simulink model "powersupply_1jan_old_top"  (R2015b)
settings: Solver=ode45  StartTime=0.0  StopTime=20*T_mach  MaxStep=4e-7  MinStep=1e-8  RelTol=1e-3
values from neighbouring files (symbols this model uses):
  c2_val = (1-V_ref/Vd_val)/(8*v2_ripple*l2_val*f_sw^2)    (= 0.0001)    [PowerSupplyScript.m]    (also in master_conv.m; master_conv2.m = 6.25e-07; matlab.mat = 1e-05; normal_buck_comparison.m = 1e-05)
  Cs = (Cs_min + Cs_max) / 2    (= 1.43223295455e-05)    [PowerSupplyScript.m]    (also in QdSnubber.m = (Cs_min + Cs_max) / 2; master_conv2.m = 3.126125e-05; matlab.mat = 2.98407954545e-05)
  delay_load = t1    (= 6e-06)    [PowerSupplyScript.m]    (also in master_conv.m; master_conv2.m; matlab.mat)
  delayVC = 2e-3    (= 0.002)    [PowerSupplyScript.m]    (also in master_conv.m = 0.001; master_conv2.m = 0; matlab.mat = 0)
  den_c1 =     [matlab.mat]
  den_c2 =     [matlab.mat]
  duty_inv = 100 - duty    (= 90)    [PowerSupplyScript.m]    (also in master_conv.m; master_conv2.m; matlab.mat)
  duty_load = (t2-t1)/T_mach*100    (= 7)    [PowerSupplyScript.m]    (also in master_conv.m; master_conv2.m; matlab.mat)
  f_sw = 50e3    (= 50000)    [PowerSupplyScript.m]    (also in master_conv.m; master_conv2.m; matlab.mat)
  frq_dc = 50    [master_conv2.m]    (also in matlab.mat = 10)
  I_ref = 10    [PowerSupplyScript.m]    (also in master_conv.m; master_conv2.m; matlab.mat)
  l1_val = Vo1*(Vd_val-Vo1)/(delta_i1*f_sw*Vd_val)    (= 0.00181818181818)    [PowerSupplyScript.m]    (also in master_conv.m = 0.000181818181818; master_conv2.m; matlab.mat; poles_locus.m = l1_val_bak)
  l2_val = 2.5*r_val*(Vd_val-V_ref)/(f_sw*Vd_val)    (= 1.36363636364e-05)    [PowerSupplyScript.m]    (also in master_conv.m; master_conv2.m = 0.00218181818182; matlab.mat = 0.002; poles_locus.m = l2_val_bak)
  num_c1 =     [matlab.mat]
  num_c2 =     [matlab.mat]
  r_val = 1    [PowerSupplyScript.m]    (also in master_conv.m; master_conv2.m; matlab.mat)
  rc2_val = 0.0001    [PowerSupplyScript.m]    (also in master_conv.m; master_conv2.m; matlab.mat)
  rl1_val = 0.0002    [PowerSupplyScript.m]    (also in master_conv.m; master_conv2.m; matlab.mat)
  rl2_val = 0.0001    [PowerSupplyScript.m]    (also in master_conv.m; master_conv2.m; matlab.mat)
  Rs = V_ref / I_ref    (= 8)    [PowerSupplyScript.m]    (also in QdSnubber.m = V_ref / I_ref; master_conv2.m; matlab.mat)
  t2 = duty * T_mach / 100    (= 2e-05)    [PowerSupplyScript.m]    (also in master_conv.m; master_conv2.m; matlab.mat)
  T_mach = 200e-6    (= 0.0002)    [PowerSupplyScript.m]    (also in master_conv.m; master_conv2.m; matlab.mat)
  V_ref = 80    [PowerSupplyScript.m]    (also in master_conv.m; master_conv2.m; matlab.mat)
  Vd_val = 110    [PowerSupplyScript.m]    (also in master_conv.m; master_conv2.m; matlab.mat)
libraries: powerlib x86, simulink x10, powerlib_meascontrol x8, simulink_extras x6
(part 2 of 2)

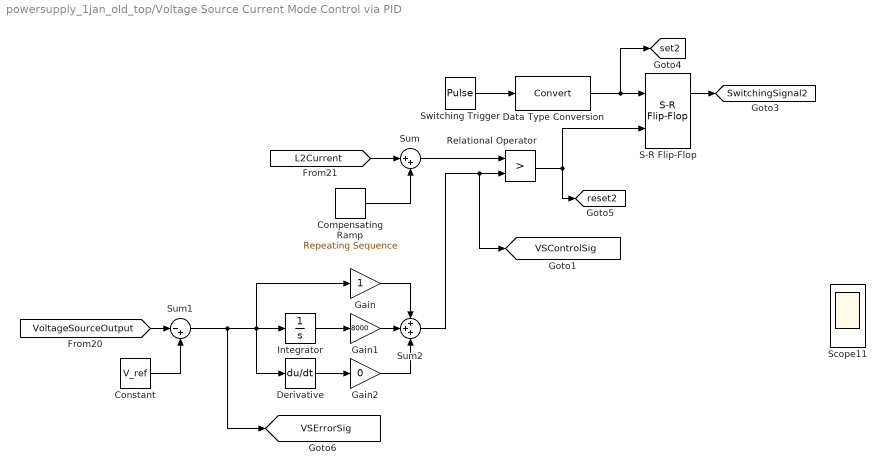
== system powersupply_1jan_old_top/Voltage Source Current Mode Control via PID ==
  Compensating Ramp : simulink/Sources/Repeating Sequence  rep_seq_t=[0 1/f_sw]  rep_seq_y=[0 80]
  Constant : Constant  Value=V_ref
  Data Type Conversion : DataTypeConversion
  Derivative : Derivative
  Gain : Gain
  Gain1 : Gain  Gain=8000
  Gain2 : Gain  Gain=0
  Integrator : Integrator
  Relational Operator : RelationalOperator  Operator=>  OutDataTypeStr=boolean
  S-R Flip-Flop : simulink_extras/Flip Flops/S-R Flip-Flop  initial_condition=0
  Scope11 : Scope  NumInputPorts=4
  Sum : Sum  Inputs=|++
  Sum1 : Sum  Inputs=|-+
  Sum2 : Sum  Inputs=+++
  Switching Trigger : DiscretePulseGenerator  PulseType=Time based  Period=1/f_sw  PulseWidth=5
  tag scope: SwitchingSignal2=global, VSControlSig=global, VSErrorSig=global, reset2=global, set2=global
  wires:
  Switching Trigger/1 -> Data Type Conversion/1
  Data Type Conversion/1 -> S-R Flip-Flop/1, [set2]
  Relational Operator/1 -> S-R Flip-Flop/2, [reset2]
  S-R Flip-Flop/1 -> [SwitchingSignal2]
  [L2Current] -> Sum/1
  Compensating Ramp/1 -> Sum/2
  Sum/1 -> Relational Operator/1
  [VoltageSourceOutput] -> Sum1/1
  Constant/1 -> Sum1/2
  Sum1/1 -> [VSErrorSig], Derivative/1, Gain/1, Integrator/1
  Integrator/1 -> Gain1/1
  Gain1/1 -> Sum2/2
  Gain/1 -> Sum2/1
  Sum2/1 -> [VSControlSig], Relational Operator/2
  Derivative/1 -> Gain2/1
  Gain2/1 -> Sum2/3

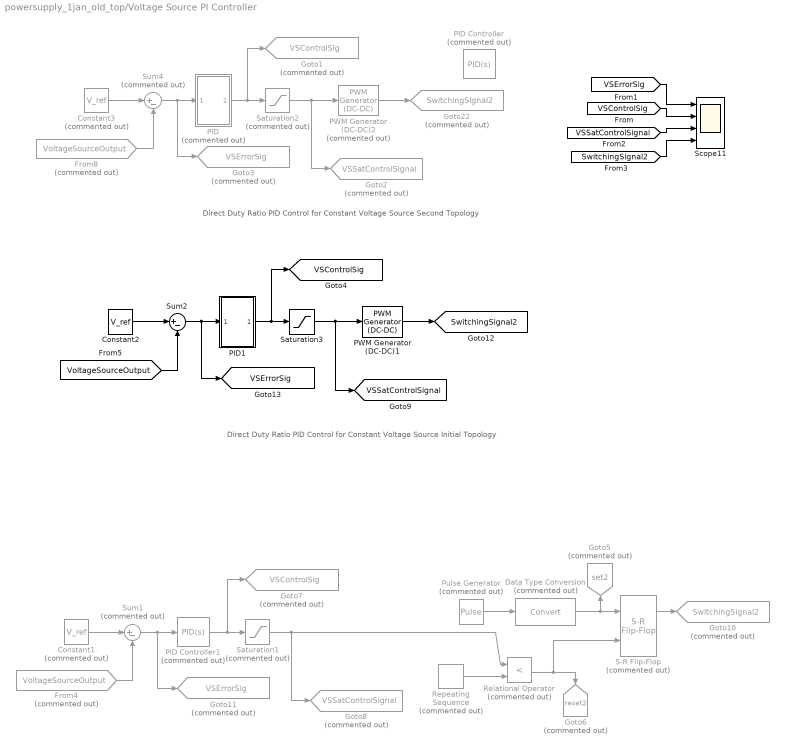
== system powersupply_1jan_old_top/Voltage Source PI Controller ==
  note: Direct Duty Ratio PID Control for Constant Voltage Source
      | Second Topology
  note: Direct Duty Ratio PID Control for Constant Voltage Source
      | Initial Topology
  Constant1 : Constant  Commented=on  Value=V_ref
  Constant2 : Constant  Value=V_ref
  Constant3 : Constant  Commented=on  Value=V_ref
  Data Type Conversion : DataTypeConversion  Commented=on
  From4 : From  Commented=on  GotoTag=VoltageSourceOutput  TagVisibility=global
  From8 : From  Commented=on  GotoTag=VoltageSourceOutput  TagVisibility=global
  Goto1 : Goto  Commented=on  GotoTag=VSControlSig  TagVisibility=global
  Goto10 : Goto  Commented=on  GotoTag=SwitchingSignal2  TagVisibility=global
  Goto11 : Goto  Commented=on  GotoTag=VSErrorSig  TagVisibility=global
  Goto2 : Goto  Commented=on  GotoTag=VSSatControlSignal  TagVisibility=global
  Goto22 : Goto  Commented=on  GotoTag=SwitchingSignal2  TagVisibility=global
  Goto3 : Goto  Commented=on  GotoTag=VSErrorSig  TagVisibility=global
  Goto5 : Goto  Commented=on  GotoTag=set2  TagVisibility=global
  Goto6 : Goto  Commented=on  GotoTag=reset2  TagVisibility=global
  Goto7 : Goto  Commented=on  GotoTag=VSControlSig  TagVisibility=global
  Goto8 : Goto  Commented=on  GotoTag=VSSatControlSignal  TagVisibility=global
  PID : Subsystem  Commented=on
  PID Controller : simulink/Continuous/PID Controller  Commented=on  Controller=PID  TimeDomain=Continuous-time  SampleTime=-1  IntegratorMethod=Forward Euler  FilterMethod=Forward Euler  Form=Parallel  UseFilter=on  ControllerParametersSource=internal  P=5  I=0  D=1  N=100000  InitialConditionSource=internal  InitialConditionForIntegrator=0  InitialConditionForFilter=0  ExternalReset=none  LimitOutput=off  UpperSaturationLimit=inf  LowerSaturationLimit=-inf  LinearizeAsGain=on  AntiWindupMode=none  Kb=1  TrackingMode=off  Kt=1  PParamMin=[]  PParamMax=[]  IParamMin=[]  IParamMax=[]  DParamMin=[]  DParamMax=[]  NParamMin=[]  NParamMax=[]  KbParamMin=[]  KbParamMax=[]  KtParamMin=[]  KtParamMax=[]  POutMin=[]  POutMax=[]  IOutMin=[]  IOutMax=[]  DOutMin=[]  DOutMax=[]  NOutMin=[]  NOutMax=[]  KbOutMin=[]  KbOutMax=[]  KtOutMin=[]  KtOutMax=[]  IntegratorOutMin=[]  IntegratorOutMax=[]  FilterOutMin=[]  FilterOutMax=[]  SumOutMin=[]  SumOutMax=[]  SumI1OutMin=[]  SumI1OutMax=[]  SumI2OutMin=[]  SumI2OutMax=[]  SumI3OutMin=[]  SumI3OutMax=[]  SumDOutMin=[]  SumDOutMax=[]  SaturationOutMin=[]  SaturationOutMax=[]  IntegratorContinuousStateAttributes=''  IntegratorStateMustResolveToSignalObject=off  IntegratorRTWStateStorageClass=Auto  FilterContinuousStateAttributes=''  FilterStateMustResolveToSignalObject=off  FilterRTWStateStorageClass=Auto  DifferentiatorICPrevScaledInput=0  DifferentiatorOutMin=[]  DifferentiatorOutMax=[]
  PID Controller1 : simulink/Continuous/PID Controller  Commented=on  Controller=PID  TimeDomain=Continuous-time  SampleTime=-1  IntegratorMethod=Forward Euler  FilterMethod=Forward Euler  Form=Parallel  UseFilter=on  ControllerParametersSource=internal  P=0.0189788446035745  I=203.066732311021  D=4.39436806782284e-07  N=6149446.46601847  InitialConditionSource=internal  InitialConditionForIntegrator=0  InitialConditionForFilter=0  ExternalReset=none  LimitOutput=off  UpperSaturationLimit=inf  LowerSaturationLimit=-inf  LinearizeAsGain=on  AntiWindupMode=none  Kb=1  TrackingMode=off  Kt=1  PParamMin=[]  PParamMax=[]  IParamMin=[]  IParamMax=[]  DParamMin=[]  DParamMax=[]  NParamMin=[]  NParamMax=[]  KbParamMin=[]  KbParamMax=[]  KtParamMin=[]  KtParamMax=[]  POutMin=[]  POutMax=[]  IOutMin=[]  IOutMax=[]  DOutMin=[]  DOutMax=[]  NOutMin=[]  NOutMax=[]  KbOutMin=[]  KbOutMax=[]  KtOutMin=[]  KtOutMax=[]  IntegratorOutMin=[]  IntegratorOutMax=[]  FilterOutMin=[]  FilterOutMax=[]  SumOutMin=[]  SumOutMax=[]  SumI1OutMin=[]  SumI1OutMax=[]  SumI2OutMin=[]  SumI2OutMax=[]  SumI3OutMin=[]  SumI3OutMax=[]  SumDOutMin=[]  SumDOutMax=[]  SaturationOutMin=[]  SaturationOutMax=[]  IntegratorContinuousStateAttributes=''  IntegratorStateMustResolveToSignalObject=off  IntegratorRTWStateStorageClass=Auto  FilterContinuousStateAttributes=''  FilterStateMustResolveToSignalObject=off  FilterRTWStateStorageClass=Auto  DifferentiatorICPrevScaledInput=0  DifferentiatorOutMin=[]  DifferentiatorOutMax=[]
  PID1 : Subsystem
  PWM Generator (DC-DC)1 : powerlib_meascontrol/Pulse & Signal Generators/PWM Generator (DC-DC)  Fsw=f_sw  Ts=0
  PWM Generator (DC-DC)2 : powerlib_meascontrol/Pulse & Signal Generators/PWM Generator (DC-DC)  Commented=on  Fsw=f_sw  Ts=0
  Pulse Generator : DiscretePulseGenerator  Commented=on  PulseType=Time based  Period=1/f_sw  PulseWidth=5
  Relational Operator : RelationalOperator  Commented=on  Operator=<  OutDataTypeStr=boolean
  Repeating Sequence : simulink/Sources/Repeating Sequence  Commented=on  rep_seq_t=[0 1/f_sw]  rep_seq_y=[0 1]
  S-R Flip-Flop : simulink_extras/Flip Flops/S-R Flip-Flop  Commented=on  initial_condition=0
  Saturation1 : Saturate  Commented=on  UpperLimit=0.99  LowerLimit=0
  Saturation2 : Saturate  Commented=on  UpperLimit=0.99  LowerLimit=0
  Saturation3 : Saturate  UpperLimit=0.99  LowerLimit=0
  Scope11 : Scope  NumInputPorts=4
  Sum1 : Sum  Commented=on  Inputs=|+-
  Sum2 : Sum  Inputs=|+-
  Sum4 : Sum  Commented=on  Inputs=|+-
  tag scope: SwitchingSignal2=global, VSControlSig=global, VSErrorSig=global, VSSatControlSignal=global
  wires:
  Constant3/1 -> Sum4/1
  From8/1 -> Sum4/2
  Saturation2/1 -> Goto2/1, PWM Generator (DC-DC)2/1
  PWM Generator (DC-DC)2/1 -> Goto22/1
  [VSErrorSig] -> Scope11/1
  [SwitchingSignal2] -> Scope11/4
  [VSSatControlSignal] -> Scope11/3
  [VSControlSig] -> Scope11/2
  Pulse Generator/1 -> Data Type Conversion/1
  Data Type Conversion/1 -> S-R Flip-Flop/1, Goto5/1
  Relational Operator/1 -> S-R Flip-Flop/2, Goto6/1
  S-R Flip-Flop/1 -> Goto10/1
  Saturation1/1 -> Goto8/1, Relational Operator/1
  Sum1/1 -> Goto11/1, PID Controller1/1
  Constant1/1 -> Sum1/1
  From4/1 -> Sum1/2
  PID Controller1/1 -> Goto7/1, Saturation1/1
  Repeating Sequence/1 -> Relational Operator/2
  Sum4/1 -> PID/1(In1), Goto3/1
  PID/1(Out1) -> Goto1/1, Saturation2/1
  Constant2/1 -> Sum2/1
  [VoltageSourceOutput] -> Sum2/2
  Saturation3/1 -> [VSSatControlSignal], PWM Generator (DC-DC)1/1
  PWM Generator (DC-DC)1/1 -> [SwitchingSignal2]
  Sum2/1 -> PID1/1(In1), [VSErrorSig]
  PID1/1(Out1) -> [VSControlSig], Saturation3/1

== system powersupply_1jan_old_top/Voltage Source PI Controller/PID ==
  In1 : Inport
  Derivative : Derivative
  Gain : Gain  Gain=2
  Gain1 : Gain  Gain=0
  Gain2 : Gain  Gain=0.0001
  Integrator : Integrator
  Sum : Sum  Inputs=+++
  Out1 : Outport
  wires:
  Gain/1 -> Sum/1
  In1/1 -> Gain/1, Integrator/1, Derivative/1
  Gain2/1 -> Sum/3
  Gain1/1 -> Sum/2
  Integrator/1 -> Gain1/1
  Derivative/1 -> Gain2/1
  Sum/1 -> Out1/1

== system powersupply_1jan_old_top/Voltage Source PI Controller/PID1 ==
  In1 : Inport
  Derivative : Derivative
  Gain : Gain
  Gain1 : Gain  Gain=60
  Gain2 : Gain  Gain=0
  Integrator : Integrator
  Sum : Sum  Inputs=+++
  Out1 : Outport
  wires:
  Gain/1 -> Sum/1
  In1/1 -> Gain/1, Integrator/1, Derivative/1
  Gain2/1 -> Sum/3
  Gain1/1 -> Sum/2
  Integrator/1 -> Gain1/1
  Derivative/1 -> Gain2/1
  Sum/1 -> Out1/1
